simulink model "UARTReadLineCSVWrite"  (R2020a)
settings: Solver=FixedStepDiscrete  StartTime=0.0  StopTime=10.0  FixedStep=1e-3  RelTol=1e-3
libraries: mbed_lib x5
settings Model: Creator=oh  LastModifiedBy=oh
settings DataIOCC: ReturnWorkspaceOutputs=off
settings OptimizationCC: DefaultParameterBehavior=Inlined  EnhancedBackFolding=on  PassReuseOutputArgsAs=Individual arguments  ZeroExternalMemoryAtStartup=off  ZeroInternalMemoryAtStartup=off  OptimizeBlockOrder=speed  DifferentSizesBufferReuse=on  OptimizationCustomize=off  EfficientTunableParamExpr=on
settings DebuggingCC: ParameterTunabilityLossMsg=error  ArithmeticOperatorsInVariantConditions=warning
settings HardwareCC: ProdBitPerPointer=32  ProdBitPerSizeT=32  ProdBitPerPtrDiffT=32  ProdLargestAtomicInteger=Long  ProdLargestAtomicFloat=Double  ProdWordSize=32  ProdHWDeviceType=ARM Compatible->ARM Cortex
settings SFSimCC: SimUseLocalCustomCode=off  MATLABDynamicMemAlloc=off  CustomCodeUndefinedFunction=UseInterfaceOnly
settings RTWCC: Description=MbedTarget (Embedded Target for Embedded Coder)  SystemTargetFile=mbed_ert.tlc  TemplateMakefile=mbed_ert.tmf  RTWUseLocalCustomCode=off  IncludeHyperlinkInReport=on  TargetLang=C++
settings CodeAppCC: ForceParamTrailComments=on  IgnoreCustomStorageClasses=off  OperatorAnnotations=on  SimulinkDataObjDesc=on  SFDataObjDesc=on  InsertBlockDesc=on
settings STFCustomTargetCC: TargetLibSuffix=.a  TargetLangStandard=C++03 (ISO)  MultiwordLength=256  GenerateSampleERTMain=on  CombineOutputUpdateFcns=on  ERTCustomFileBanners=on  SupportContinuousTime=off  SupportNonInlinedSFcns=off  RemoveResetFunc=on  MATLABClassNameForMDSCustomization=Simulink.SoftwareTarget.ERTCustomization  ModelStepFunctionPrototypeControlCompliant=on  SystemTargetFile=mbed_ert.tlc
settings ERTTargetCC: TargetLangStandard=C++03 (ISO)  GenerateSampleERTMain=on  ParMdlRefBuildCompliant=off  CompOptLevelCompliant=off  ConcurrentExecutionCompliant=off  CPPClassGenCompliant=off  UseToolchainInfoCompliant=off  InlinedParameterPlacement=NonHierarchical  ERTCustomFileTemplate=mbed_ert_file_process.tlc

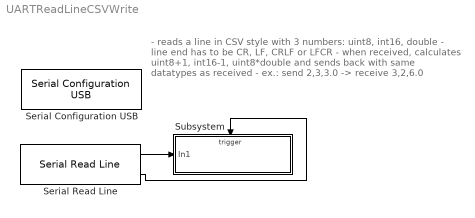
== system UARTReadLineCSVWrite ==
  note: - reads a line in CSV style with 3 numbers: uint8, int16, double
      | - line end has to be CR, LF, CRLF or LFCR
      | - when received,
      |     calculates uint8+1, int16-1, uint8*double
      |     and sends back with same datatypes as received
      | - ex.: send 2,3,3.0 -> receive 3,2,6.0
  Serial Configuration USB : mbed_lib/Serial/UART/Serial Configuration USB  Priority=0  BaudRate=115200
      settings: SourceProductName=Mbed Target
  Serial Read Line : mbed_lib/Serial/UART/Serial Read Line  SerialPort=USB  NumDataPort=off  NewDataPort=on  BufferSize=100  SampleTime=0.1
      settings: SourceProductName=Mbed Target
  Subsystem : Subsystem
  wires:
  Serial Read Line/1 -> Subsystem/1(In1)
  Serial Read Line/2 -> Subsystem/Trigger

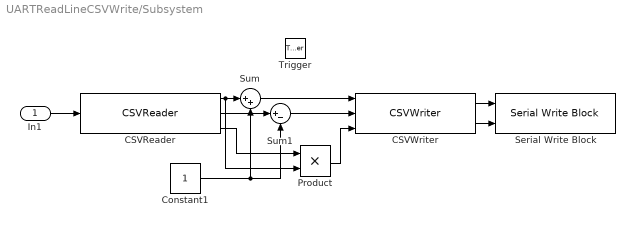
== system UARTReadLineCSVWrite/Subsystem ==
  In1 : Inport  OutDataTypeStr=uint8
  Trigger : TriggerPort  VariantControl=Variant  PortDimensions=1
  CSVReader : mbed_lib/Utilities/CSVReader  TypeOutputPorts={ 'uint8' 1 'int16' 1 'double' 1 }  TypeOfOutputs={'1*uint8' '1*int16' '1*double'}  BufferSize=0  SampleTime=-1
      settings: SourceProductName=Mbed Target
  CSVWriter : mbed_lib/Utilities/CSVWriter  TypeInputPorts={ 'uint8' 1 'int16' 1 'double' 1 }  TypeOfInputs={'1*uint8' '1*int16' '1*double'}  BufferSize=100  errEn=off  SampleTime=-1
      settings: SourceProductName=Mbed Target
  Constant1 : Constant  OutDataTypeStr=Inherit: Inherit via back propagation
  Product : Product
  Serial Write Block : mbed_lib/Serial/UART/Serial Write Block  SerialPort=USB  numData=on  SampleTime=-1
      settings: SourceProductName=Mbed Target
  Sum : Sum  Inputs=|++  OutDataTypeStr=uint8
  Sum1 : Sum  Inputs=|+-  OutDataTypeStr=int16
  wires:
  CSVWriter/1 -> Serial Write Block/1
  CSVWriter/2 -> Serial Write Block/2
  In1/1 -> CSVReader/1
  CSVReader/1 -> Product/2, Sum/1
  Sum1/1 -> CSVWriter/2
  Sum/1 -> CSVWriter/1
  CSVReader/2 -> Sum1/1
  Constant1/1 -> Sum/2, Sum1/2
  Product/1 -> CSVWriter/3
  CSVReader/3 -> Product/1
